simulink model "One_Sensor_Simulation"  (R2021a)
settings: Solver=FixedStepAuto  StartTime=0.0  StopTime=200  FixedStep=Ts  RelTol=1e-5
values from neighbouring files (symbols this model uses):
  accel_filter_coef = [    0.0264    0.1405    0.3331    0.3331    0.1405    0.0264]    [quad_params_ekf.m]
  g = ref_acc(3)    [ekf_measurement_jacobian.m]    (also in quad_params_ekf.m = 9.81)
  gyro_filter_den = [ 1.0000    2.2287    2.5245    1.5773    0.5410    0.0796]    [quad_params_ekf.m]
  gyro_filter_num = [ 0.2821    1.2725    2.4208    2.4208    1.2725    0.2821]    [quad_params_ekf.m]
  I = [     0.005831943165131                   0                   0 ... (first row only)    [quad_params_ekf.m]
  Kd_rates = [0.05,0.05,0.1]'    [quad_params_ekf.m]
  Kd_vel = [0.8,0.8,0.3]'    [quad_params_ekf.m]
  Ki_vel = [0.1,0.1,0.1]'    [quad_params_ekf.m]
  km = 1.2e-7    (= 1.2e-07)    [quad_params_ekf.m]
  Kp_att = [6,6,6]'    [quad_params_ekf.m]
  Kp_pos = [7,7,3]'    [quad_params_ekf.m]
  Kp_rates = [10,10,10]'    [quad_params_ekf.m]
  Kp_vel = [3,3,5]'    [quad_params_ekf.m]
  kt = 0.9e-5    (= 9e-06)    [quad_params_ekf.m]
  L = 0.2    [quad_params_ekf.m]
  m = 0.9272    [quad_params_ekf.m]
  q_init = [1;0;0;0]    [quad_params_ekf.m]
  rate_p_max = 3.5    [quad_params_ekf.m]
  thrust_max = thrust_max_per_motor*4    (= 32)    [quad_params_ekf.m]
  thrust_max_per_motor = 8    [quad_params_ekf.m]
  tilt_max = pi/6    (= 0.523598775598)    [quad_params_ekf.m]
  TQ_max_per_motor = km*(w_max.^2)    [quad_params_ekf.m]
  Ts = 0.001    [ekf_process_jacobian.m]    (also in ekf_process_model.m; quad_params_ekf.m)
  Ts_IMU = 0.001    [quad_params_ekf.m]
  Vb_init = [0;0;0]    [quad_params_ekf.m]
  vel_xy_max = 15    [quad_params_ekf.m]
  vel_z_max = 10    [quad_params_ekf.m]
  wb_init = [0;0;0]    [quad_params_ekf.m]
  Xe_init = [0;0;0]    [quad_params_ekf.m]
undefined symbols (not defined in the file or in its folder): IMU, pm_0, sigbuilder_block, Vm_0, xme_0
libraries: simulink_extras x7, aerolibutil x6, sharedutil x5, simulink x4, sharedtransform x4, pid_lib x3, aerolibcommonsys x3, aerolibnavsys x2, mspsensorlib x1, aerolibnav x1, aerolibanim x1
(part 1 of 3)
settings Model: Creator=Petronas-Tareq  LastModifiedBy=Petronas-Tareq
settings SolverCC: AutoInsertRateTranBlk=on  InsertRTBMode=Always

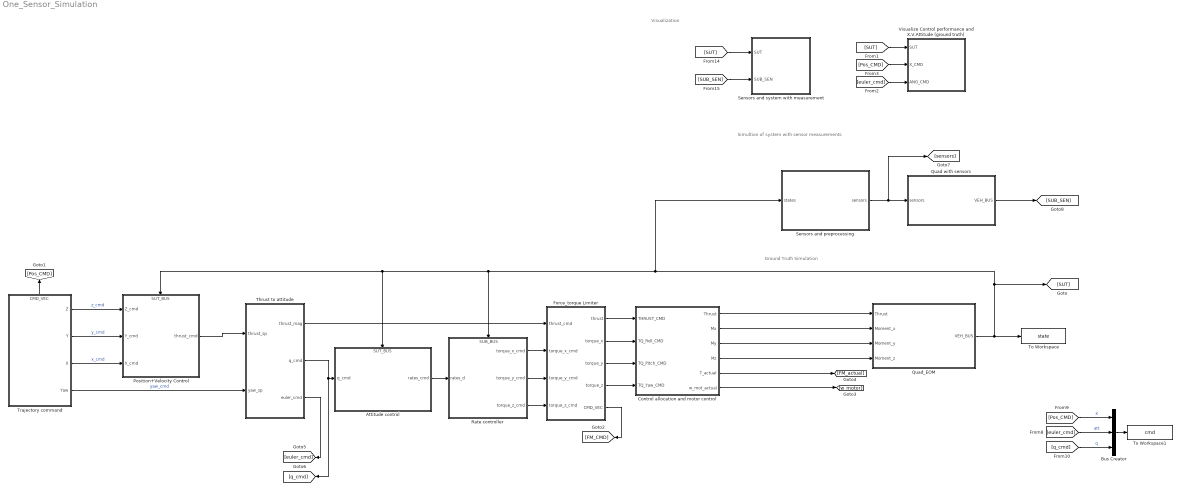
== system One_Sensor_Simulation ==
  note: Ground Truth Simulation
  note: Simultion of system with sensor measurements
  note: Visualization
  Attitude control : Subsystem
      settings: PortSchema="{\"entries\":[{\"content\":{\"sides\":[{\"content\":{\"connectorIds\":[\"In1\"]},\"type\":\"ConnectorPlacement.EquallySpacedRectSide\",\"uuid\":\"19a574f6-5314-4727-8968-5b1c9712010e\"},{\"content\":{\"connectorIds\":[\"Out1\"],\"side\":\"RIGHT\"},\"type\":\"ConnectorPlacement.EquallySpacedRectSide\",\"uuid\":\"5cd6813f-6e17-48c1-918b-7c366c6d9cfa\"},{\"content\":{\"connectorIds\":[\"In2\"],\"side\":\"TOP\"},\"type\":\"ConnectorPlacement.EquallySpacedRectSide\",\"uuid\":\"b2bca67c-c4f4-4722-89a0-a16251073bfd\"}]},\"type\":\"ConnectorPlacement.EquallySpacedConnector\",\"uuid\":\"dcbf54f5-c136-40d5-a3db-9d2776e5196c\"}],\"packageUris\":[\"http://schema.mathworks.com/mf0/Connector/R2020b\"],\"version\":\"1.0\"}"
      mask Display: image('$imagefile'); % Use "Edit Image" on toolstrip to change.
  Bus Creator : BusCreator  Inputs=3
  Control allocation and motor control : Subsystem  Variant=on  VariantControlMode=label  LabelModeActiveChoice=Choice1
      mask Display: image('$imagefile'); % Use "Edit Image" on toolstrip to change.
  Force_torque Limiter : Subsystem
  Position+Velocity Control : Subsystem
      settings: PortSchema="{\"entries\":[{\"content\":{\"sides\":[{\"content\":{\"connectorIds\":[\"In1\",\"In2\",\"In3\"]},\"type\":\"ConnectorPlacement.EquallySpacedRectSide\",\"uuid\":\"cfe37ea9-b8e2-443a-9d65-596f0fda79c9\"},{\"content\":{\"connectorIds\":[\"Out1\"],\"side\":\"RIGHT\"},\"type\":\"ConnectorPlacement.EquallySpacedRectSide\",\"uuid\":\"f39f64e1-4b16-444a-b7d2-95ecb1b2a6fa\"},{\"content\":{\"connectorIds\":[\"In4\"],\"side\":\"TOP\"},\"type\":\"ConnectorPlacement.EquallySpacedRectSide\",\"uuid\":\"52402c3a-f2ac-44cf-8c94-dbfc3f851d2b\"}]},\"type\":\"ConnectorPlacement.EquallySpacedConnector\",\"uuid\":\"0122f56a-2702-493b-af7d-a25e6b9e04ed\"}],\"packageUris\":[\"http://schema.mathworks.com/mf0/Connector/R2020b\"],\"version\":\"1.0\"}"
  Quad with sensors : Subsystem
      mask Display: image('$imagefile'); % Use "Edit Image" on toolstrip to change.
  Quad_EOM : Subsystem
      mask Display: image('$imagefile'); % Use "Edit Image" on toolstrip to change.
  Rate controller : Subsystem
      settings: PortSchema="{\"entries\":[{\"content\":{\"sides\":[{\"content\":{\"connectorIds\":[\"In1\"]},\"type\":\"ConnectorPlacement.EquallySpacedRectSide\",\"uuid\":\"0af60e35-7b10-4750-a6af-1a3d920b4771\"},{\"content\":{\"connectorIds\":[\"Out1\",\"Out2\",\"Out3\"],\"side\":\"RIGHT\"},\"type\":\"ConnectorPlacement.EquallySpacedRectSide\",\"uuid\":\"931b0f34-b3f1-4a41-949f-3d763eca3151\"},{\"content\":{\"connectorIds\":[\"In2\"],\"side\":\"TOP\"},\"type\":\"ConnectorPlacement.EquallySpacedRectSide\",\"uuid\":\"84fe42fa-07d1-4fd9-ad2f-8c6651eaa98c\"}]},\"type\":\"ConnectorPlacement.EquallySpacedConnector\",\"uuid\":\"f603d2ac-5c20-4a82-ba8b-1c7971d6778a\"}],\"packageUris\":[\"http://schema.mathworks.com/mf0/Connector/R2020b\"],\"version\":\"1.0\"}"
  Sensors and preprocessing : Subsystem
  Sensors and system with measurement : Subsystem
  Thrust to attitude : Subsystem
  To Workspace : ToWorkspace  VariableName=state  SaveFormat=Timeseries  SampleTime=-1
  To Workspace1 : ToWorkspace  VariableName=cmd  SaveFormat=Timeseries  SampleTime=-1
  Trajectory command : Subsystem  Variant=on  VariantControlMode=label  LabelModeActiveChoice=5
      settings: PortSchema="{\"entries\":[{\"content\":{\"sides\":[{\"content\":{\"connectorIds\":[]},\"type\":\"ConnectorPlacement.EquallySpacedRectSide\",\"uuid\":\"8b658e99-682c-4d99-9859-63a6cdcf875c\"},{\"content\":{\"connectorIds\":[\"Out1\",\"Out2\",\"Out3\",\"Out4\"],\"side\":\"RIGHT\"},\"type\":\"ConnectorPlacement.EquallySpacedRectSide\",\"uuid\":\"566e7e32-52b1-45cc-9bb3-5343461c1cc0\"},{\"content\":{\"connectorIds\":[\"Out5\"],\"side\":\"TOP\"},\"type\":\"ConnectorPlacement.EquallySpacedRectSide\",\"uuid\":\"4cb1ab19-6483-4408-b5f4-106b35038f17\"}]},\"type\":\"ConnectorPlacement.EquallySpacedConnector\",\"uuid\":\"dc7c82fc-432d-4c18-9829-e6c2b483f5a7\"}],\"packageUris\":[\"http://schema.mathworks.com/mf0/Connector/R2020b\"],\"version\":\"1.0\"}"
  Visualize Control performance and X,V,Attitude (ground truth) : Subsystem
  wires:
  Force_torque Limiter/5(CMD_VEC) -> [FM_CMD]
  Trajectory command/2(Y) -> Position+Velocity Control/2(Y_cmd)  "y_cmd"
  [SUT] -> Visualize Control performance and X,V,Attitude (ground truth)/1(SUT)
  [Pos_CMD] -> Visualize Control performance and X,V,Attitude (ground truth)/2(X_CMD)
  Trajectory command/3(X) -> Position+Velocity Control/3(X_cmd)  "x_cmd"
  Control allocation and motor control/1(Thrust) -> Quad_EOM/1(Thrust)
  Control allocation and motor control/2(Mx) -> Quad_EOM/2(Moment_x)
  Control allocation and motor control/3(My) -> Quad_EOM/3(Moment_y)
  Control allocation and motor control/4(Mz) -> Quad_EOM/4(Moment_z)
  Control allocation and motor control/5(T_actual) -> [FM_actual]
  Control allocation and motor control/6(w_mot_actual) -> [w_motor]
  Trajectory command/1(Z) -> Position+Velocity Control/1(Z_cmd)  "z_cmd"
  [euler_cmd] -> Visualize Control performance and X,V,Attitude (ground truth)/3(ANG_CMD)
  Force_torque Limiter/4(torque_z) -> Control allocation and motor control/4(TQ_Yaw_CMD)
  Force_torque Limiter/3(torque_y) -> Control allocation and motor control/3(TQ_Pitch_CMD)
  Force_torque Limiter/2(torque_x) -> Control allocation and motor control/2(TQ_Roll_CMD)
  Force_torque Limiter/1(thrust) -> Control allocation and motor control/1(THRUST_CMD)
  Thrust to attitude/1(thrust_mag) -> Force_torque Limiter/1(thrust_cmd)
  Rate controller/2(torque_y_cmd) -> Force_torque Limiter/3(torque_y_cmd)
  Rate controller/3(torque_z_cmd) -> Force_torque Limiter/4(torque_z_cmd)
  Rate controller/1(torque_x_cmd) -> Force_torque Limiter/2(torque_x_cmd)
  Attitude control/1(rates_cmd) -> Rate controller/1(rates_d)
  Trajectory command/5(CMD_VEC) -> [Pos_CMD]
  Bus Creator/1 -> To Workspace1/1
  [Pos_CMD] -> Bus Creator/1  "X"
  [euler_cmd] -> Bus Creator/2  "att"
  [q_cmd] -> Bus Creator/3  "q"
  Thrust to attitude/2(q_cmd) -> Attitude control/1(q_cmd), [q_cmd]
  Thrust to attitude/3(euler_cmd) -> [euler_cmd]
  Trajectory command/4(Yaw) -> Thrust to attitude/2(yaw_sp)  "yaw_cmd"
  Position+Velocity Control/1(thrust_cmd) -> Thrust to attitude/1(thrust_sp)
  Quad_EOM/1(VEH_BUS) -> Position+Velocity Control/4(SUT_BUS), Attitude control/2(SUT_BUS), Rate controller/2(SUB_BUS), Sensors and preprocessing/1(states), [SUT], To Workspace/1
  Sensors and preprocessing/1(sensors) -> [sensors], Quad with sensors/1(sensors)
  Quad with sensors/1(VEH_BUS) -> [SUB_SEN]
  [SUT] -> Sensors and system with measurement/1(SUT)
  [SUB_SEN] -> Sensors and system with measurement/2(SUB_SEN)

== system One_Sensor_Simulation/Attitude control ==
  note: Attitude control (full attitude control, i.e. yaw+thrust)
  note: Attitude Error Calculation
  q_cmd : Inport
  SUT_BUS : Inport  Port=2
  Bus Selector3 : BusSelector  OutputSignals=q
  K_attitude : Gain  Gain=Kp_att
  MATLAB Function1 : MATLAB Function  TreatAsAtomicUnit=on
  Product : Product
  Quaternion Inverse : aerolibutil/Quaternion Inverse
  Quaternion multiply : aerolibutil/Quaternion Multiplication
  Selector1 : Selector  InputPortWidth=4  IndexOptions=Index vector (dialog)  Indices=1  OutputSizes=1
  Selector2 : Selector  InputPortWidth=4  IndexOptions=Index vector (dialog)  Indices=2:4  OutputSizes=1
  k : Gain  Gain=2
  rates_cmd : Outport  VectorParamsAs1DForOutWhenUnconnected=off
  wires:
  SUT_BUS/1 -> [SUT]
  q_cmd/1 -> Quaternion multiply/2  "q_d"
  [SUT] -> Bus Selector3/1
  Bus Selector3/1 -> Quaternion Inverse/1  "<q>"
  Product/1 -> k/1  "error"
  Selector1/1 -> MATLAB Function1/1(q0)  "q0"
  MATLAB Function1/1(y) -> Product/1
  Selector2/1 -> Product/2  "q_vec"
  Quaternion multiply/1 -> Selector2/1, Selector1/1  "qe"
  k/1 -> K_attitude/1
  Quaternion Inverse/1 -> Quaternion multiply/1
  K_attitude/1 -> rates_cmd/1  "rates_cmd"

== system One_Sensor_Simulation/Control allocation and motor control ==
  note: 1) Add Subsystem or Model blocks as valid variant choices.
      | 2) You cannot connect blocks at this level. At simulation, connectivity is automatically
      | determined, based on the active variant and port name matching.
  THRUST_CMD : Inport
  TQ_Roll_CMD : Inport  Port=2
  TQ_Pitch_CMD : Inport  Port=3
  TQ_Yaw_CMD : Inport  Port=4
  Ideal Actuators with allocation : Subsystem  VariantControl=Choice2
  Ideal Actuattion (direct transfer) : Subsystem  VariantControl=Choice1
  Thrust : Outport
  Mx : Outport  Port=2
  My : Outport  Port=3
  Mz : Outport  Port=4
  T_actual : Outport  Port=5
  w_mot_actual : Outport  Port=6

== system One_Sensor_Simulation/Force_torque Limiter ==
  thrust_cmd : Inport
  torque_x_cmd : Inport  Port=2
  torque_y_cmd : Inport  Port=3
  torque_z_cmd : Inport  Port=4
  Mux : Mux
  Saturation : Saturate  UpperLimit=thrust_max  LowerLimit=-thrust_max
      settings: AttributesFormatString=|
      | MAX =    %<UpperLimit>
      | MIN = %<LowerLimit>
  Saturation1 : Saturate  UpperLimit=2*TQ_max_per_motor  LowerLimit=-2*TQ_max_per_motor
      settings: AttributesFormatString=|
      | MAX =    %<UpperLimit>
      | MIN = %<LowerLimit>
  Saturation2 : Saturate  UpperLimit=thrust_max_per_motor*L  LowerLimit=-thrust_max_per_motor *L
      settings: AttributesFormatString=|
      | MAX =    %<UpperLimit>
      | MIN = %<LowerLimit>
  Saturation3 : Saturate  UpperLimit=thrust_max_per_motor*L  LowerLimit=-thrust_max_per_motor *L
      settings: AttributesFormatString=|
      | MAX =    %<UpperLimit>
      | MIN = %<LowerLimit>
  Scope : Scope
  thrust : Outport  VectorParamsAs1DForOutWhenUnconnected=off
  torque_x : Outport  Port=2  VectorParamsAs1DForOutWhenUnconnected=off
  torque_y : Outport  Port=3  VectorParamsAs1DForOutWhenUnconnected=off
  torque_z : Outport  Port=4  VectorParamsAs1DForOutWhenUnconnected=off
  CMD_VEC : Outport  Port=5  VectorParamsAs1DForOutWhenUnconnected=off
  wires:
  torque_z_cmd/1 -> Saturation1/1
  thrust_cmd/1 -> Saturation/1
  torque_y_cmd/1 -> Saturation2/1
  torque_x_cmd/1 -> Saturation3/1
  Saturation/1 -> [THRUST], thrust/1
  Saturation3/1 -> [TQ_Roll_X], torque_x/1
  Saturation2/1 -> [TQ_Pitch_Y], torque_y/1
  Saturation1/1 -> [TQ_Yaw_Z], torque_z/1
  Mux/1 -> Scope/1, CMD_VEC/1
  [THRUST] -> Mux/1
  [TQ_Roll_X] -> Mux/2
  [TQ_Pitch_Y] -> Mux/3
  [TQ_Yaw_Z] -> Mux/4

== system One_Sensor_Simulation/Position+Velocity Control ==
  note: Velocity PID controller
  note: Position P controller
  Z_cmd : Inport
  Y_cmd : Inport  Port=2
  X_cmd : Inport  Port=3
  SUT_BUS : Inport  Port=4
  Bus Selector3 : BusSelector  OutputSignals=Xe,Ve
  Mux : Mux  Inputs=3
  Position P Controller : Subsystem
  To Workspace2 : ToWorkspace  VariableName=thrust_sp  SaveFormat=Timeseries  SampleTime=-1
  Velocity PID Controller : Subsystem
  acc setpoint : Constant  Value=[0;0;0]
  thrust_cmd : Outport
  wires:
  SUT_BUS/1 -> [SUT]
  [SUT] -> Bus Selector3/1
  Bus Selector3/1 -> [P]  "<Xe>"
  Mux/1 -> [P_sp]
  acc setpoint/1 -> [acc_sp]
  [acc_sp] -> Velocity PID Controller/3(acc_ff)  "acc_feedforwad"
  Position P Controller/1(V_sp) -> Velocity PID Controller/1(vel_cmd)  "vel_cmd"
  [P_sp] -> Position P Controller/1(pos_cmd)
  [P] -> Position P Controller/2(pos_cur)
  [V] -> Velocity PID Controller/2(vel_cur)
  Velocity PID Controller/1(thrust_sp) -> To Workspace2/1, thrust_cmd/1  "thrust_cmd"
  Bus Selector3/2 -> [V]  "<Ve>"
  Z_cmd/1 -> Mux/3
  X_cmd/1 -> Mux/1
  Y_cmd/1 -> Mux/2

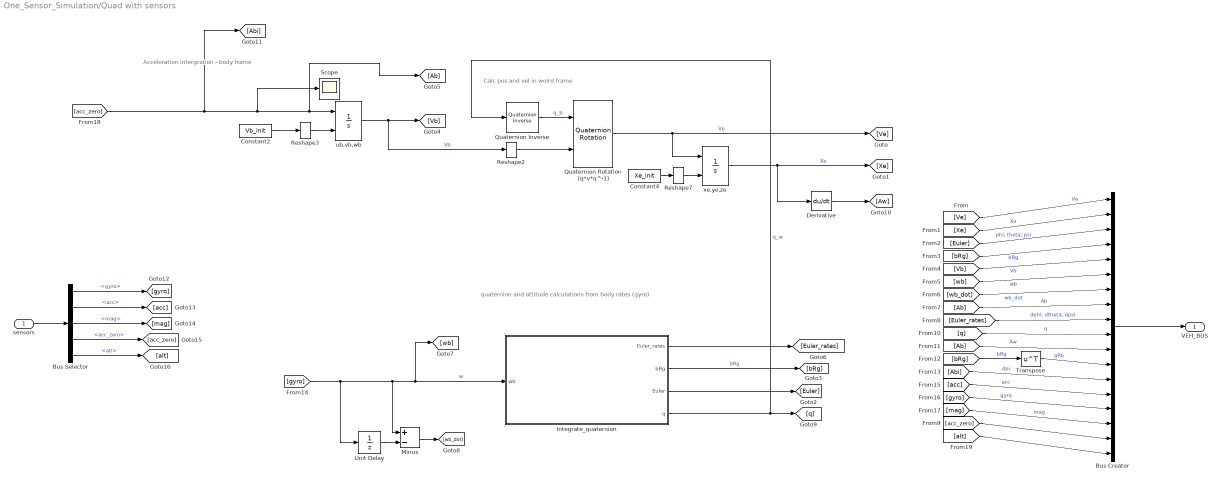
== system One_Sensor_Simulation/Quad with sensors ==
  note: Acceleration intergration - body frame
  note: Calc pos and vel in wolrd frame
  note: quaternion and attitude calculations from body rates (gyro)
  sensors : Inport
  Bus Creator : BusCreator  Inputs=18
  Bus Selector : BusSelector  OutputSignals=gyro,acc,mag,acc_zero,alt
  Constant2 : Constant  Value=Vb_init  OutDataTypeStr=Inherit: Inherit via back propagation
  Constant4 : Constant  Value=Xe_init  OutDataTypeStr=Inherit: Inherit via back propagation
  Derivative : Derivative
  Integrate_quaternion : Subsystem
  Minus : Sum  Inputs=+-
  Quaternion Inverse : aerolibutil/Quaternion Inverse
  Quaternion Rotation (q*v*q^-1) : aerolibutil/Quaternion Rotation
  Reshape2 : Reshape  OutputDimensionality=Column vector (2-D)
  Reshape3 : Reshape  OutputDimensionality=Column vector (2-D)
  Reshape7 : Reshape  OutputDimensionality=Column vector (2-D)
  Scope : Scope
  Transpose : Math  Operator=transpose  SaturateOnIntegerOverflow=on
  Unit Delay : UnitDelay  SampleTime=-1  HasFrameUpgradeWarning=on
  ub,vb,wb : Integrator  InitialConditionSource=external  InitialCondition=Vm_0
  xe,ye,ze : Integrator  InitialConditionSource=external  InitialCondition=xme_0
  VEH_BUS : Outport  VectorParamsAs1DForOutWhenUnconnected=off
  wires:
  [Euler] -> Bus Creator/3  "phi; theta; psi"
  [Xe] -> Bus Creator/2  "Xe"
  [Ve] -> Bus Creator/1  "Ve"
  [bRg] -> Bus Creator/4  "bRg"
  [Ab] -> Bus Creator/8  "Ab"
  [wb_dot] -> Bus Creator/7  "wb_dot"
  Bus Creator/1 -> VEH_BUS/1
  [Vb] -> Bus Creator/5  "Vb"
  [wb] -> Bus Creator/6  "wb"
  [Euler_rates] -> Bus Creator/9  "dphi; dtheta; dpsi"
  Constant2/1 -> Reshape3/1
  Integrate_quaternion/2(bRg) -> [bRg]  "bRg"
  Constant4/1 -> Reshape7/1
  Reshape3/1 -> ub,vb,wb/2
  Reshape7/1 -> xe,ye,ze/2
  Quaternion Rotation (q*v*q^-1)/1 -> xe,ye,ze/1, [Ve]  "Ve"
  xe,ye,ze/1 -> Derivative/1, [Xe]  "Xe"
  [gyro] -> Unit Delay/1, Minus/1, Integrate_quaternion/1(wb), [wb]  "w"
  ub,vb,wb/1 -> [Vb], Reshape2/1  "Vb"
  Integrate_quaternion/1(Euler_rates) -> [Euler_rates]
  Integrate_quaternion/3(Euler) -> [Euler]
  [q] -> Bus Creator/10  "q"
  Integrate_quaternion/4(q) -> Quaternion Inverse/1, [q]  "q_w"
  Reshape2/1 -> Quaternion Rotation (q*v*q^-1)/2
  Quaternion Inverse/1 -> Quaternion Rotation (q*v*q^-1)/1  "q_b"
  Derivative/1 -> [Aw]
  [Ab] -> Bus Creator/11  "Aw"
  [bRg] -> Transpose/1  "bRg"
  Transpose/1 -> Bus Creator/12  "gRb"
  [Abi] -> Bus Creator/13  "Abi"
  Unit Delay/1 -> Minus/2
  Minus/1 -> [wb_dot]
  Bus Selector/1 -> [gyro]  "<gyro>"
  Bus Selector/2 -> [acc]  "<acc>"
  sensors/1 -> Bus Selector/1
  [acc_zero] -> [Abi], Scope/1, [Ab], ub,vb,wb/1
  [acc] -> Bus Creator/14  "acc"
  [gyro] -> Bus Creator/15  "gyro"
  Bus Selector/3 -> [mag]  "<mag>"
  [mag] -> Bus Creator/16  "mag"
  Bus Selector/4 -> [acc_zero]  "<acc_zero>"
  [acc_zero] -> Bus Creator/17
  Bus Selector/5 -> [alt]  "<alt>"
  [alt] -> Bus Creator/18

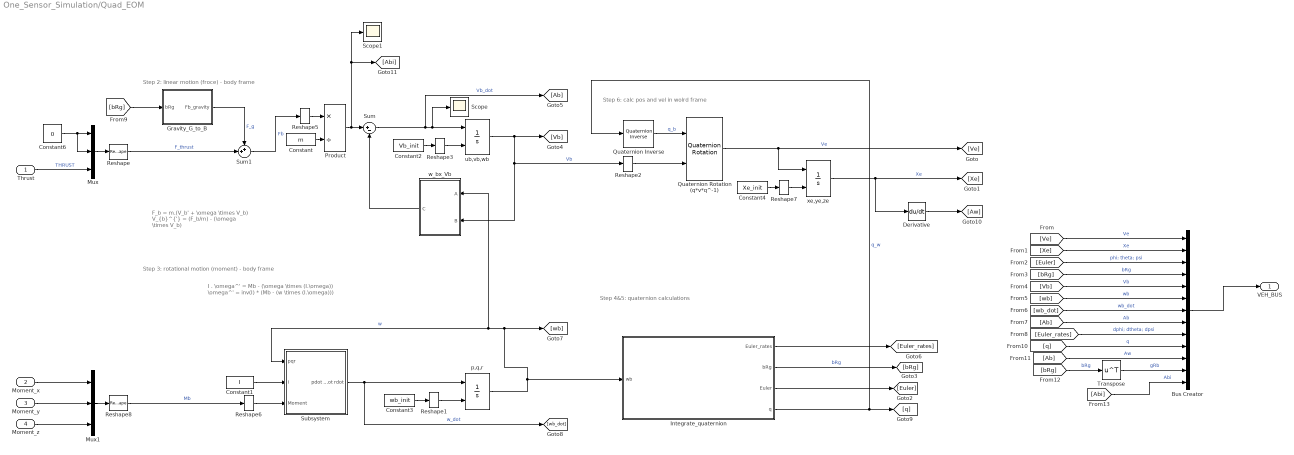
== system One_Sensor_Simulation/Quad_EOM ==
  note: Step 3: rotational motion (moment) - body frame
  note: F_b = m.(V_b' + \omega \times V_b)
      |
      | V_{b}^{'} = (F_b/m) - (\omega \times V_b)
  note: Step 2: linear motion (froce) - body frame
  note: Step 6: calc pos and vel in wolrd frame
  note: I . \omega^' = Mb - (\omega \times (I.\omega))
      |
      | \omega^' = inv(I) * (Mb - (w \times (I.\omega)))
  note: Step 4&5: quaternion calculations
  Thrust : Inport
  Moment_x : Inport  Port=2
  Moment_y : Inport  Port=3
  Moment_z : Inport  Port=4
  Bus Creator : BusCreator  Inputs=13
  Constant : Constant  Value=m  OutDataTypeStr=Inherit: Inherit via back propagation
  Constant1 : Constant  Value=I  OutDataTypeStr=Inherit: Inherit via back propagation
  Constant2 : Constant  Value=Vb_init  OutDataTypeStr=Inherit: Inherit via back propagation
  Constant3 : Constant  Value=wb_init  OutDataTypeStr=Inherit: Inherit via back propagation
  Constant4 : Constant  Value=Xe_init  OutDataTypeStr=Inherit: Inherit via back propagation
  Constant6 : Constant  Value=0
  Derivative : Derivative
  Gravity_G_to_B : Subsystem
  Integrate_quaternion : Subsystem
  Mux : Mux  Inputs=3
  Mux1 : Mux  Inputs=3
  Product : Product  Inputs=*/  SaturateOnIntegerOverflow=on  OutDataTypeStr=Inherit: Same as first input
  Quaternion Inverse : aerolibutil/Quaternion Inverse
  Quaternion Rotation (q*v*q^-1) : aerolibutil/Quaternion Rotation
  Reshape{,1..3,5..8} (8 alike) : Reshape  OutputDimensionality=Column vector (2-D)
  Scope : Scope
  Scope1 : Scope
  Subsystem : Subsystem
  Sum : Sum  Inputs=|+-  SaturateOnIntegerOverflow=on
  Sum1 : Sum  Inputs=++|
  Transpose : Math  Operator=transpose  SaturateOnIntegerOverflow=on
  "p,q,r " : Integrator  InitialConditionSource=external  InitialCondition=pm_0
  ub,vb,wb : Integrator  InitialConditionSource=external  InitialCondition=Vm_0
  w_bx_Vb : Subsystem
      mask Display:
      | text(.5,.5,'Cross\nProduct\n\nC = AxB', ...
      | 	'HorizontalAlignment','Center',...
      | 	'VerticalAlignment','middle')
  xe,ye,ze : Integrator  InitialConditionSource=external  InitialCondition=xme_0
  VEH_BUS : Outport  VectorParamsAs1DForOutWhenUnconnected=off
  wires:
  [Euler] -> Bus Creator/3  "phi; theta; psi"
  [Xe] -> Bus Creator/2  "Xe"
  [Ve] -> Bus Creator/1  "Ve"
  [bRg] -> Bus Creator/4  "bRg"
  [Ab] -> Bus Creator/8  "Ab"
  [wb_dot] -> Bus Creator/7  "wb_dot"
  Bus Creator/1 -> VEH_BUS/1
  [Vb] -> Bus Creator/5  "Vb"
  [wb] -> Bus Creator/6  "wb"
  [Euler_rates] -> Bus Creator/9  "dphi; dtheta; dpsi"
  Reshape8/1 -> Reshape6/1  "Mb"
  Reshape6/1 -> Subsystem/3(Moment)
  Reshape1/1 -> "p,q,r "/2
  Constant2/1 -> Reshape3/1
  Subsystem/1(pdot qdot rdot) -> [wb_dot], "p,q,r "/1  "w_dot"
  Constant/1 -> Product/2
  Constant1/1 -> Subsystem/2(I)
  w_bx_Vb/1(C) -> Sum/2
  Integrate_quaternion/2(bRg) -> [bRg]  "bRg"
  Sum/1 -> [Ab], Scope/1, ub,vb,wb/1  "Vb_dot"
  Constant4/1 -> Reshape7/1
  Reshape3/1 -> ub,vb,wb/2
  Reshape7/1 -> xe,ye,ze/2
  Quaternion Rotation (q*v*q^-1)/1 -> xe,ye,ze/1, [Ve]  "Ve"
  Reshape5/1 -> Product/1
  xe,ye,ze/1 -> Derivative/1, [Xe]  "Xe"
  Sum1/1 -> Reshape5/1  "Fb"
  Constant3/1 -> Reshape1/1
  Product/1 -> Scope1/1, [Abi], Sum/1
  Constant6/1 -> Mux/2, Mux/1
  Gravity_G_to_B/1(Fb_gravity) -> Sum1/1  "F_g"
  Mux/1 -> Reshape/1
  Reshape/1 -> Sum1/2  "F_thrust"
  Thrust/1 -> Mux/3  "THRUST"
  [bRg] -> Gravity_G_to_B/1(bRg)
  Moment_y/1 -> Mux1/2
  Moment_z/1 -> Mux1/3
  Mux1/1 -> Reshape8/1
  Moment_x/1 -> Mux1/1
  "p,q,r "/1 -> [wb], Subsystem/1(pqr), w_bx_Vb/1(A), Integrate_quaternion/1(wb)  "w"
  ub,vb,wb/1 -> [Vb], Reshape2/1, w_bx_Vb/2(B)  "Vb"
  Integrate_quaternion/1(Euler_rates) -> [Euler_rates]
  Integrate_quaternion/3(Euler) -> [Euler]
  [q] -> Bus Creator/10  "q"
  Integrate_quaternion/4(q) -> Quaternion Inverse/1, [q]  "q_w"
  Reshape2/1 -> Quaternion Rotation (q*v*q^-1)/2
  Quaternion Inverse/1 -> Quaternion Rotation (q*v*q^-1)/1  "q_b"
  Derivative/1 -> [Aw]
  [Ab] -> Bus Creator/11  "Aw"
  [bRg] -> Transpose/1  "bRg"
  Transpose/1 -> Bus Creator/12  "gRb"
  [Abi] -> Bus Creator/13  "Abi"

== system One_Sensor_Simulation/Rate controller ==
  note: Rate controller
  rates_d : Inport
  SUB_BUS : Inport  Port=2
  Bus Selector1 : BusSelector  OutputSignals=wb,wb_dot
  Demux : Demux  Outputs=3
  Kd_rates : Gain  Gain=Kd_rates
  Kp_rates : Gain  Gain=Kp_rates
  Scope : Scope  NumInputPorts=2
  Sum : Sum  Inputs=|+-
  Sum1 : Sum  Inputs=|+-
  limit rate p : Saturate  UpperLimit=rate_p_max  LowerLimit=-rate_p_max
  limit rate q : Saturate  UpperLimit=rate_p_max  LowerLimit=-rate_p_max
  limit rate r : Saturate  UpperLimit=rate_p_max  LowerLimit=-rate_p_max
  torque_x_cmd : Outport
  torque_y_cmd : Outport  Port=2
  torque_z_cmd : Outport  Port=3
  wires:
  Bus Selector1/2 -> Kd_rates/1  "<wb_dot>"
  Bus Selector1/1 -> Sum1/2, Scope/2  "<wb>"
  Demux/1 -> limit rate p/1
  Demux/2 -> limit rate q/1
  Demux/3 -> limit rate r/1
  SUB_BUS/1 -> Bus Selector1/1  "measurements"
  rates_d/1 -> Sum1/1, Scope/1
  Kd_rates/1 -> Sum/2  "w_d"
  Kp_rates/1 -> Sum/1
  Sum/1 -> Demux/1  "torques"
  Sum1/1 -> Kp_rates/1
  limit rate p/1 -> torque_x_cmd/1
  limit rate q/1 -> torque_y_cmd/1
  limit rate r/1 -> torque_z_cmd/1

== system One_Sensor_Simulation/Sensors and preprocessing ==
  states : Inport
  Bus Creator4 : BusCreator  Inputs=5
  IMU+altitude : Subsystem
  Memory1 : Memory  InheritSampleTime=on
  Preprocessing and Filtering : Subsystem
  Scope : Scope
  Scope1 : Scope
  sensors : Outport
  wires:
  states/1 -> Memory1/1
  Bus Creator4/1 -> sensors/1
  IMU+altitude/1(acc) -> Scope/1, Preprocessing and Filtering/1(acc_raw)  "acc_raw"
  IMU+altitude/2(gyro) -> Scope1/1, Preprocessing and Filtering/2(gyro_raw)  "gyro_raw"
  Memory1/1 -> IMU+altitude/1(States)
  IMU+altitude/3(alt) -> Preprocessing and Filtering/3(alt_raw)  "alt_raw"
  IMU+altitude/4(mag) -> Preprocessing and Filtering/4(mag_raw)  "mag_raw"
  Preprocessing and Filtering/1(acc_zero) -> Bus Creator4/1  "acc_zero"
  Preprocessing and Filtering/2(acc) -> Bus Creator4/2  "acc"
  Preprocessing and Filtering/3(gyro) -> Bus Creator4/3  "gyro"
  Preprocessing and Filtering/4(alt) -> Bus Creator4/4  "alt"
  Preprocessing and Filtering/5(mag) -> Bus Creator4/5  "mag"

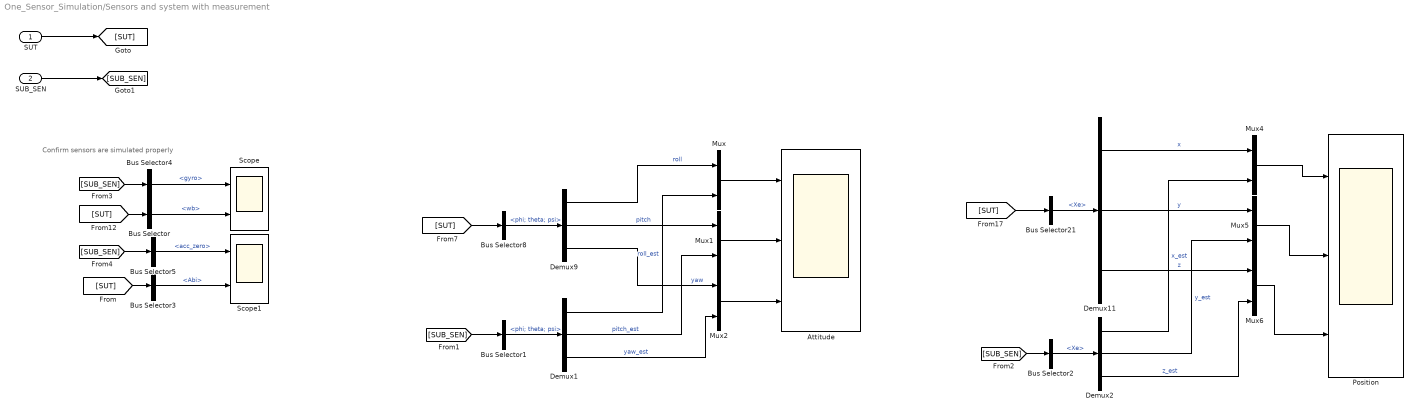
== system One_Sensor_Simulation/Sensors and system with measurement ==
  note: Confirm sensors are simulated properly
  SUT : Inport
  SUB_SEN : Inport  Port=2
  "Attitude " : Scope  NumInputPorts=3
  Bus Selector : BusSelector  OutputSignals=wb
  Bus Selector1 : BusSelector  OutputSignals=phi; theta; psi
  Bus Selector2 : BusSelector  OutputSignals=Xe
  Bus Selector21 : BusSelector  OutputSignals=Xe
  Bus Selector3 : BusSelector  OutputSignals=Abi
  Bus Selector4 : BusSelector  OutputSignals=gyro
  Bus Selector5 : BusSelector  OutputSignals=acc_zero
  Bus Selector8 : BusSelector  OutputSignals=phi; theta; psi
  Demux{1..2,9,11} (4 alike) : Demux  Outputs=3
  Mux{,1..2,4..6} (6 alike) : Mux  Inputs=2
  Position : Scope  NumInputPorts=3
  Scope : Scope  NumInputPorts=2
  Scope1 : Scope  NumInputPorts=2
  wires:
  Mux4/1 -> Position/1
  Demux11/2 -> Mux5/1  "y"
  [SUT] -> Bus Selector21/1
  Demux11/1 -> Mux4/1  "x"
  Mux5/1 -> Position/2
  Demux11/3 -> Mux6/1  "z"
  Bus Selector21/1 -> Demux11/1  "<Xe>"
  [SUT] -> Bus Selector8/1
  Mux6/1 -> Position/3
  Bus Selector8/1 -> Demux9/1  "<phi; theta; psi>"
  Mux2/1 -> "Attitude "/3
  Demux9/2 -> Mux1/1  "pitch"
  Demux9/3 -> Mux2/1  "yaw"
  Mux1/1 -> "Attitude "/2
  Mux/1 -> "Attitude "/1
  Demux9/1 -> Mux/1  "roll"
  SUT/1 -> [SUT]
  SUB_SEN/1 -> [SUB_SEN]
  [SUB_SEN] -> Bus Selector1/1
  Bus Selector1/1 -> Demux1/1  "<phi; theta; psi>"
  Demux1/1 -> Mux/2  "roll_est"
  Demux1/2 -> Mux1/2  "pitch_est"
  Demux1/3 -> Mux2/2  "yaw_est"
  [SUB_SEN] -> Bus Selector2/1
  Bus Selector2/1 -> Demux2/1  "<Xe>"
  Demux2/1 -> Mux4/2  "x_est"
  Demux2/2 -> Mux5/2  "y_est"
  Demux2/3 -> Mux6/2  "z_est"
  Bus Selector/1 -> Scope/2  "<wb>"
  Bus Selector4/1 -> Scope/1  "<gyro>"
  Bus Selector5/1 -> Scope1/1  "<acc_zero>"
  [SUT] -> Bus Selector3/1
  [SUB_SEN] -> Bus Selector4/1
  [SUB_SEN] -> Bus Selector5/1
  [SUT] -> Bus Selector/1
  Bus Selector3/1 -> Scope1/2  "<Abi>"

== system One_Sensor_Simulation/Thrust to attitude ==
  note: Thrust vector and Yaw to Attitude and total Thrust
  thrust_sp : Inport
  yaw_sp : Inport  Port=2
  Bus Creator : BusCreator  Inputs=3
  Demux4 : Demux  Outputs=3
  Direction Cosine Matrix to Quaternions : sharedtransform/Direction Cosine Matrix  to Quaternions  aMode=0  action=None  tolerance=eps(2)
      settings: SourceProductBaseCode=AE,PW,DR,MT,UV,VE
  MATLAB Function4 : MATLAB Function  TreatAsAtomicUnit=on
  Quaternions to Rotation Angles : sharedtransform/Quaternions to Rotation Angles  rotationOrder=ZYX  aMode=aMode
      settings: SourceProductBaseCode=AE,PW,DR,MT,UV,VE
  Scope1 : Scope
  Scope2 : Scope
  To Workspace : ToWorkspace  VariableName=thrust_unit_dir  SaveFormat=Timeseries  SampleTime=-1
  To Workspace1 : ToWorkspace  VariableName=thrust_mag  SaveFormat=Timeseries  SampleTime=-1
  thrust_mag : Outport
  q_cmd : Outport  Port=2
  euler_cmd : Outport  Port=3
  wires:
  thrust_sp/1 -> Scope1/1, MATLAB Function4/1(thrust_sp)  "thrust_cmd"
  MATLAB Function4/1(R_sp) -> To Workspace/1, Direction Cosine Matrix to Quaternions/1
  MATLAB Function4/2(thrust_mag) -> thrust_mag/1, To Workspace1/1
  Direction Cosine Matrix to Quaternions/1 -> q_cmd/1, Quaternions to Rotation Angles/1
  yaw_sp/1 -> MATLAB Function4/2(yaw_sp)  "yaw_cmd"
  Demux4/1 -> Bus Creator/1  "yaw"
  Demux4/3 -> Bus Creator/3  "roll"
  Bus Creator/1 -> Scope2/1, euler_cmd/1
  Demux4/2 -> Bus Creator/2  "pitch"
  Quaternions to Rotation Angles/1 -> Demux4/1

== system One_Sensor_Simulation/Trajectory command ==
  Altitude : Subsystem  VariantControl=1
  Ground : Subsystem  VariantControl=0
  Position Trajectory : Subsystem  VariantControl=5
  Test to visualize thrust dir : Subsystem  VariantControl=6
  X Sine : Subsystem  VariantControl=4
  X ramp : Subsystem  VariantControl=9
  X square : Subsystem  VariantControl=7
  Y Sine : Subsystem  VariantControl=3
  Y ramp : Subsystem  VariantControl=8
  Yaw Sine : Subsystem  VariantControl=2
  Yaw steps : Subsystem  VariantControl=10
  Z : Outport
  Y : Outport  Port=2
  X : Outport  Port=3
  Yaw : Outport  Port=4
  CMD_VEC : Outport  Port=5

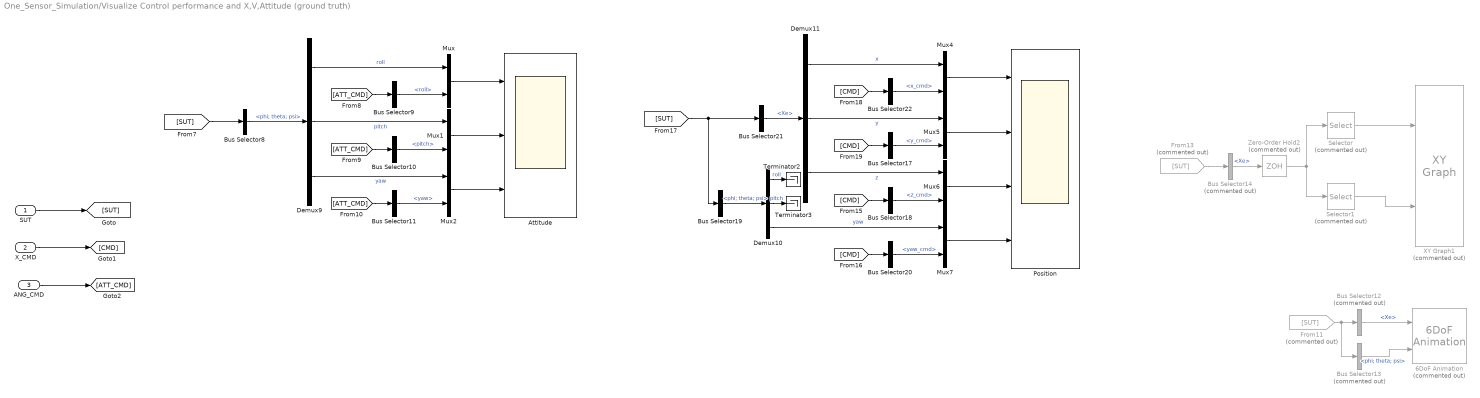
== system One_Sensor_Simulation/Visualize Control performance and X,V,Attitude (ground truth) ==
  SUT : Inport
  X_CMD : Inport  Port=2
  ANG_CMD : Inport  Port=3
  6DoF Animation : aerolibanim/6DoF Animation  Commented=on  u1=[-20 20 -20 20 -20 20]  u2=0.05  u3=0.5  u4=[-5 -5 0 5]  u5=Fly alongside  u6=[0 0 0]  u7=10  u8=on
  "Attitude " : Scope  NumInputPorts=3
  Bus Selector10 : BusSelector  OutputSignals=pitch
  Bus Selector11 : BusSelector  OutputSignals=yaw
  Bus Selector12 : BusSelector  Commented=on  OutputSignals=Xe
  Bus Selector13 : BusSelector  Commented=on  OutputSignals=phi; theta; psi
  Bus Selector14 : BusSelector  Commented=on  OutputSignals=Xe
  Bus Selector17 : BusSelector  OutputSignals=y_cmd
  Bus Selector18 : BusSelector  OutputSignals=z_cmd
  Bus Selector19 : BusSelector  OutputSignals=phi; theta; psi
  Bus Selector20 : BusSelector  OutputSignals=yaw_cmd
  Bus Selector21 : BusSelector  OutputSignals=Xe
  Bus Selector22 : BusSelector  OutputSignals=x_cmd
  Bus Selector8 : BusSelector  OutputSignals=phi; theta; psi
  Bus Selector9 : BusSelector  OutputSignals=roll
  Demux10 : Demux  Outputs=3
  Demux11 : Demux  Outputs=3
  Demux9 : Demux  Outputs=3
  From11 : From  Commented=on  GotoTag=SUT
  From13 : From  Commented=on  GotoTag=SUT
  Mux{,1..2,4..7} (7 alike) : Mux  Inputs=2
  Position : Scope  NumInputPorts=4
  Selector : Selector  Commented=on  InputPortWidth=3  IndexOptions=Index vector (dialog)  Indices=1  OutputSizes=1
  Selector1 : Selector  Commented=on  InputPortWidth=3  IndexOptions=Index vector (dialog)  Indices=2  OutputSizes=1
  Terminator2 : Terminator
  Terminator3 : Terminator
  XY Graph1 : simulink/Sinks/XY Graph  Commented=on  xmin=-1  xmax=30  ymin=-1  ymax=35  st=-1
  Zero-Order Hold2 : ZeroOrderHold  Commented=on  SampleTime=0.1
  wires:
  SUT/1 -> [SUT]
  X_CMD/1 -> [CMD]
  [SUT] -> Bus Selector8/1
  Demux9/2 -> Mux1/1  "pitch"
  Demux9/1 -> Mux/1  "roll"
  Bus Selector8/1 -> Demux9/1  "<phi; theta; psi>"
  Mux/1 -> "Attitude "/1
  Mux1/1 -> "Attitude "/2
  Mux2/1 -> "Attitude "/3
  Demux9/3 -> Mux2/1  "yaw"
  [ATT_CMD] -> Bus Selector9/1
  Bus Selector9/1 -> Mux/2  "<roll>"
  [ATT_CMD] -> Bus Selector10/1
  Bus Selector10/1 -> Mux1/2  "<pitch>"
  [ATT_CMD] -> Bus Selector11/1
  Bus Selector11/1 -> Mux2/2  "<yaw>"
  From13/1 -> Bus Selector14/1
  Bus Selector14/1 -> Zero-Order Hold2/1  "<Xe>"
  Zero-Order Hold2/1 -> Selector1/1, Selector/1
  Demux10/3 -> Mux7/1  "yaw"
  Mux7/1 -> Position/4
  Demux11/1 -> Mux4/1  "x"
  [CMD] -> Bus Selector20/1
  Bus Selector20/1 -> Mux7/2  "<yaw_cmd>"
  [CMD] -> Bus Selector17/1
  [SUT] -> Bus Selector21/1, Bus Selector19/1
  Demux10/2 -> Terminator3/1  "pitch"
  Mux6/1 -> Position/3
  Bus Selector19/1 -> Demux10/1  "<phi; theta; psi>"
  Demux10/1 -> Terminator2/1  "roll"
  Demux11/2 -> Mux5/1  "y"
  Bus Selector17/1 -> Mux5/2  "<y_cmd>"
  Mux4/1 -> Position/1
  Demux11/3 -> Mux6/1  "z"
  [CMD] -> Bus Selector22/1
  Mux5/1 -> Position/2
  Bus Selector22/1 -> Mux4/2  "<x_cmd>"
  Bus Selector18/1 -> Mux6/2  "<z_cmd>"
  [CMD] -> Bus Selector18/1
  Bus Selector21/1 -> Demux11/1  "<Xe>"
  ANG_CMD/1 -> [ATT_CMD]
  Selector/1 -> XY Graph1/1
  Selector1/1 -> XY Graph1/2
  From11/1 -> Bus Selector13/1, Bus Selector12/1
  Bus Selector12/1 -> 6DoF Animation/1  "<Xe>"
  Bus Selector13/1 -> 6DoF Animation/2  "<phi; theta; psi>"

== system One_Sensor_Simulation/Control allocation and motor control/Ideal Actuators with allocation ==
  THRUST_CMD : Inport
  TQ_Roll_CMD : Inport  Port=2
  TQ_Pitch_CMD : Inport  Port=3
  TQ_Yaw_CMD : Inport  Port=4
  Control allocation : Subsystem
  Perfect actuators : Subsystem  VariantControl=Choice2
  Thrust : Outport
  Mx : Outport  Port=2
  My : Outport  Port=3
  Mz : Outport  Port=4
  T_actual : Outport  Port=5
  w_mot_actual : Outport  Port=6
  wires:
  Control allocation/1(w_command) -> Perfect actuators/1(w_cmd)
  THRUST_CMD/1 -> Control allocation/1(THRUST_CMD)
  TQ_Pitch_CMD/1 -> Control allocation/3(TQ_Pitch_CMD)
  TQ_Roll_CMD/1 -> Control allocation/2(TQ_Roll_CMD)
  TQ_Yaw_CMD/1 -> Control allocation/4(TQ_Yaw_CMD)
  Perfect actuators/5(T_actual) -> T_actual/1
  Perfect actuators/6(w_mot_actual) -> w_mot_actual/1
  Perfect actuators/3(My) -> My/1
  Perfect actuators/2(Mx) -> Mx/1
  Perfect actuators/4(Mz) -> Mz/1
  Perfect actuators/1(Thrust) -> Thrust/1

== system One_Sensor_Simulation/Control allocation and motor control/Ideal Actuattion (direct transfer) ==
  THRUST_CMD : Inport
  TQ_Roll_CMD : Inport  Port=2
  TQ_Pitch_CMD : Inport  Port=3
  TQ_Yaw_CMD : Inport  Port=4
  Mux : Mux
  Zero : Constant  Value=[0;0;0;0]  OutDataTypeStr=Inherit: Inherit via back propagation
  Thrust : Outport
  Mx : Outport  Port=2
  My : Outport  Port=3
  Mz : Outport  Port=4
  T_actual : Outport  Port=5
  w_mot_actual : Outport  Port=6
  wires:
  Zero/1 -> w_mot_actual/1
  TQ_Pitch_CMD/1 -> Mux/3, My/1
  TQ_Roll_CMD/1 -> Mux/2, Mx/1
  TQ_Yaw_CMD/1 -> Mux/4, Mz/1
  THRUST_CMD/1 -> Mux/1, Thrust/1
  Mux/1 -> T_actual/1

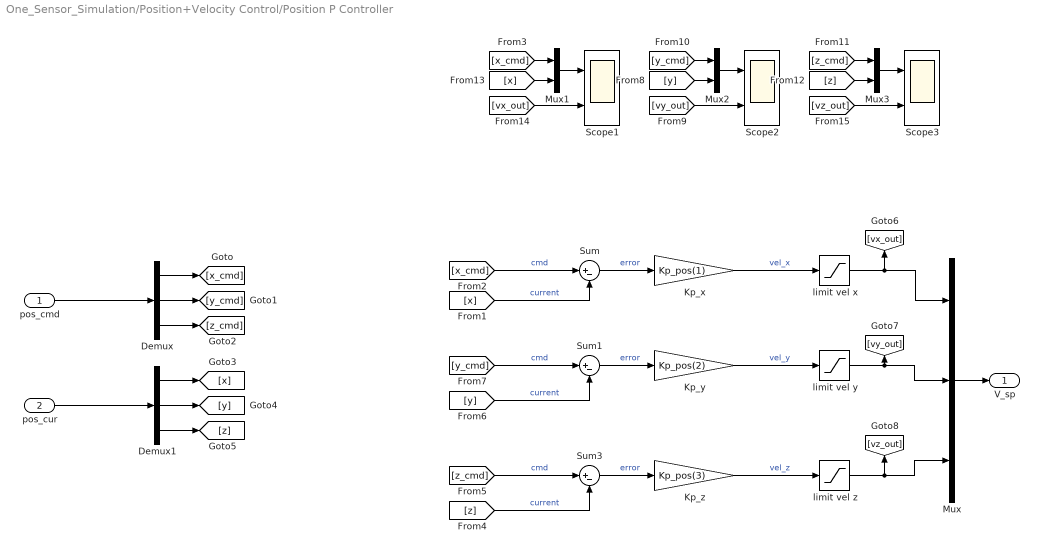
== system One_Sensor_Simulation/Position+Velocity Control/Position P Controller ==
  pos_cmd : Inport
  pos_cur : Inport  Port=2
  Demux : Demux  Outputs=3
  Demux1 : Demux  Outputs=3
  Kp_x : Gain  Gain=Kp_pos(1)
  Kp_y : Gain  Gain=Kp_pos(2)
  Kp_z : Gain  Gain=Kp_pos(3)
  Mux : Mux  Inputs=3
  Mux1 : Mux  Inputs=2
  Mux2 : Mux  Inputs=2
  Mux3 : Mux  Inputs=2
  Scope1 : Scope  NumInputPorts=2
  Scope2 : Scope  NumInputPorts=2
  Scope3 : Scope  NumInputPorts=2
  Sum : Sum  Inputs=|+-
  Sum1 : Sum  Inputs=|+-
  Sum3 : Sum  Inputs=|+-
  limit vel x : Saturate  UpperLimit=vel_xy_max  LowerLimit=-vel_xy_max
  limit vel y : Saturate  UpperLimit=vel_xy_max  LowerLimit=-vel_xy_max
  limit vel z : Saturate  UpperLimit=vel_z_max  LowerLimit=-vel_z_max
  V_sp : Outport
  wires:
  pos_cmd/1 -> Demux/1
  pos_cur/1 -> Demux1/1
  Demux/1 -> [x_cmd]
  Demux/2 -> [y_cmd]
  Demux/3 -> [z_cmd]
  Demux1/1 -> [x]
  Demux1/3 -> [z]
  Demux1/2 -> [y]
  [x_cmd] -> Sum/1  "cmd"
  Sum/1 -> Kp_x/1  "error"
  Mux/1 -> V_sp/1
  Kp_x/1 -> limit vel x/1  "vel_x"
  [x] -> Sum/2  "current"
  [z_cmd] -> Sum3/1  "cmd"
  [z] -> Sum3/2  "current"
  Sum3/1 -> Kp_z/1  "error"
  [y_cmd] -> Sum1/1  "cmd"
  [y] -> Sum1/2  "current"
  Sum1/1 -> Kp_y/1  "error"
  Kp_z/1 -> limit vel z/1  "vel_z"
  limit vel x/1 -> [vx_out], Mux/1
  Kp_y/1 -> limit vel y/1  "vel_y"
  limit vel y/1 -> [vy_out], Mux/2
  limit vel z/1 -> [vz_out], Mux/3
  [x_cmd] -> Mux1/1
  Mux1/1 -> Scope1/1
  [vx_out] -> Scope1/2
  [x] -> Mux1/2
  [y_cmd] -> Mux2/1
  Mux2/1 -> Scope2/1
  [vy_out] -> Scope2/2
  [y] -> Mux2/2
  [z_cmd] -> Mux3/1
  Mux3/1 -> Scope3/1
  [vz_out] -> Scope3/2
  [z] -> Mux3/2

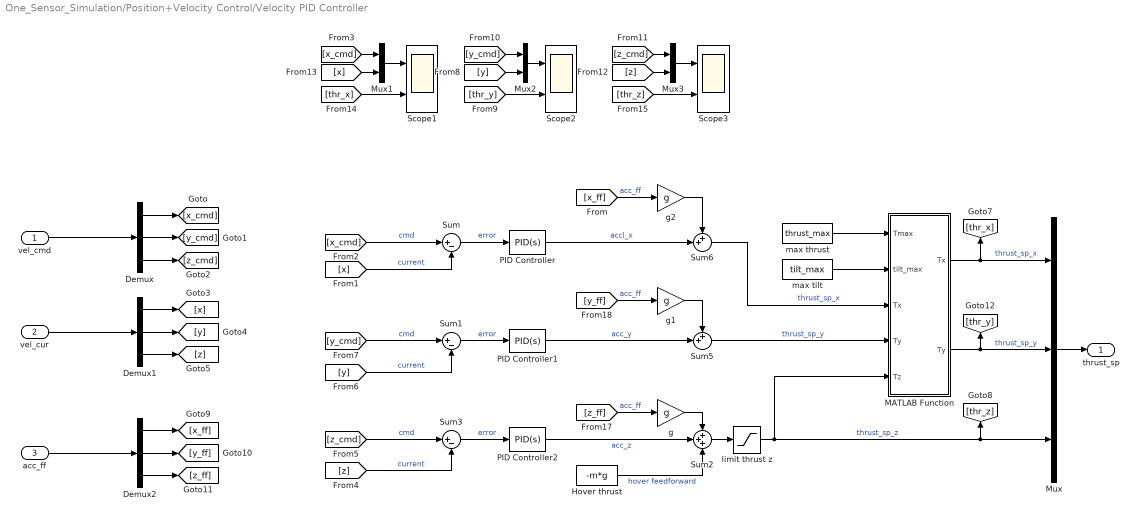
== system One_Sensor_Simulation/Position+Velocity Control/Velocity PID Controller ==
  vel_cmd : Inport
  vel_cur : Inport  Port=2
  acc_ff : Inport  Port=3
  Demux : Demux  Outputs=3
  Demux1 : Demux  Outputs=3
  Demux2 : Demux  Outputs=3
  Hover thrust : Constant  Value=-m*g
  MATLAB Function : MATLAB Function  TreatAsAtomicUnit=on
  Mux : Mux  Inputs=3
  Mux1 : Mux  Inputs=2
  Mux2 : Mux  Inputs=2
  Mux3 : Mux  Inputs=2
  PID Controller : pid_lib/PID Controller  Controller=PID  Form=Parallel  TimeDomain=Continuous-time  UseExternalTs=off  SampleTime=-1  IntegratorMethod=Forward Euler  FilterMethod=Forward Euler  ControllerParametersSource=internal  P=Kp_vel(1)  I=Ki_vel(1)  D=Kd_vel(1)  UseFilter=on  N=100  TunerSelectOption=Transfer Function Based (PID Tuner App)  InitialConditionSource=internal  InitialConditionForIntegrator=0  InitialConditionForFilter=0  DifferentiatorICPrevScaledInput=0  ExternalReset=none  TrackingMode=off  Kt=1  LimitOutput=off  SatLimitsSource=internal  UpperSaturationLimit=inf  LowerSaturationLimit=-inf  LinearizeAsGain=on  AntiWindupMode=none  Kb=1  POutMin=[]  POutMax=[]  IOutMin=[]  IOutMax=[]  DOutMin=[]  DOutMax=[]  NOutMin=[]  NOutMax=[]  SumOutMin=[]  SumOutMax=[]  SaturationOutMin=[]  SaturationOutMax=[]  PParamMin=[]  PParamMax=[]  IParamMin=[]  IParamMax=[]  DParamMin=[]  DParamMax=[]  NParamMin=[]  NParamMax=[]  KbParamMin=[]  KbParamMax=[]  KtParamMin=[]  KtParamMax=[]  KbOutMin=[]  KbOutMax=[]  KtOutMin=[]  KtOutMax=[]  IntegratorOutMin=[]  IntegratorOutMax=[]  FilterOutMin=[]  FilterOutMax=[]  SumI1OutMin=[]  SumI1OutMax=[]  SumI2OutMin=[]  SumI2OutMax=[]  SumI3OutMin=[]  SumI3OutMax=[]  SumI4OutMin=[]  SumI4OutMax=[]  SumDOutMin=[]  SumDOutMax=[]  DifferentiatorOutMin=[]  DifferentiatorOutMax=[]  FilterDiffOutCoefMin=[]  FilterDiffOutCoefMax=[]  ReciprocalOutMin=[]  ReciprocalOutMax=[]  SumDenOutMin=[]  SumDenOutMax=[]  SumNumOutMin=[]  SumNumOutMax=[]  DivideOutMin=[]  DivideOutMax=[]  UdiffTsProdOutMin=[]  UdiffTsProdOutMax=[]  NTsProdOutMin=[]  NTsProdOutMax=[]  UintegralTsProdOutMin=[]  UintegralTsProdOutMax=[]  UngainTsProdOutMin=[]  UngainTsProdOutMax=[]  IntegratorContinuousStateAttributes=''  IntegratorStateMustResolveToSignalObject=off  IntegratorRTWStateStorageClass=Auto  FilterContinuousStateAttributes=''  FilterStateMustResolveToSignalObject=off  FilterRTWStateStorageClass=Auto  ParallelPVariant=InternalParameters  IdealPVariant=Disabled  IVariant=InternalParameters  DVariant=InternalParameters  IntegratorVariant=Continuous  SatVariant=Disabled  AWVariant=Passthrough  PCopyVariant=Disabled  TRVariant=Disabled  FdbkBlocksVariant=Forward  IdealPFdbkVariant=Disabled  SatFdbkVariant=Disabled  DerivativeFilterVariant=ContFilter  NVariant=InternalParameters  NCopyVariant=Disabled  FilterICVariant=InternalICsFilter  IntegratorICVariant=InternalICs  ExternalResetVariant=Disabled  TRSumVariant=Passthrough  SumFdbkVariant=Disabled  SumVariant=Sum_PID  TsampFilterVariant=InternalTs  TsampNgainVariant=Passthrough  TsampIntegralVariant=Passthrough  ExternalSaturationOutDataTypeStr=Inherit: Same as second input
  PID Controller1 : pid_lib/PID Controller  Controller=PID  Form=Parallel  TimeDomain=Continuous-time  UseExternalTs=off  SampleTime=-1  IntegratorMethod=Forward Euler  FilterMethod=Forward Euler  ControllerParametersSource=internal  P=Kp_vel(2)  I=Ki_vel(2)  D=Kd_vel(2)  UseFilter=on  N=100  TunerSelectOption=Transfer Function Based (PID Tuner App)  InitialConditionSource=internal  InitialConditionForIntegrator=0  InitialConditionForFilter=0  DifferentiatorICPrevScaledInput=0  ExternalReset=none  TrackingMode=off  Kt=1  LimitOutput=off  SatLimitsSource=internal  UpperSaturationLimit=inf  LowerSaturationLimit=-inf  LinearizeAsGain=on  AntiWindupMode=none  Kb=1  POutMin=[]  POutMax=[]  IOutMin=[]  IOutMax=[]  DOutMin=[]  DOutMax=[]  NOutMin=[]  NOutMax=[]  SumOutMin=[]  SumOutMax=[]  SaturationOutMin=[]  SaturationOutMax=[]  PParamMin=[]  PParamMax=[]  IParamMin=[]  IParamMax=[]  DParamMin=[]  DParamMax=[]  NParamMin=[]  NParamMax=[]  KbParamMin=[]  KbParamMax=[]  KtParamMin=[]  KtParamMax=[]  KbOutMin=[]  KbOutMax=[]  KtOutMin=[]  KtOutMax=[]  IntegratorOutMin=[]  IntegratorOutMax=[]  FilterOutMin=[]  FilterOutMax=[]  SumI1OutMin=[]  SumI1OutMax=[]  SumI2OutMin=[]  SumI2OutMax=[]  SumI3OutMin=[]  SumI3OutMax=[]  SumI4OutMin=[]  SumI4OutMax=[]  SumDOutMin=[]  SumDOutMax=[]  DifferentiatorOutMin=[]  DifferentiatorOutMax=[]  FilterDiffOutCoefMin=[]  FilterDiffOutCoefMax=[]  ReciprocalOutMin=[]  ReciprocalOutMax=[]  SumDenOutMin=[]  SumDenOutMax=[]  SumNumOutMin=[]  SumNumOutMax=[]  DivideOutMin=[]  DivideOutMax=[]  UdiffTsProdOutMin=[]  UdiffTsProdOutMax=[]  NTsProdOutMin=[]  NTsProdOutMax=[]  UintegralTsProdOutMin=[]  UintegralTsProdOutMax=[]  UngainTsProdOutMin=[]  UngainTsProdOutMax=[]  IntegratorContinuousStateAttributes=''  IntegratorStateMustResolveToSignalObject=off  IntegratorRTWStateStorageClass=Auto  FilterContinuousStateAttributes=''  FilterStateMustResolveToSignalObject=off  FilterRTWStateStorageClass=Auto  ParallelPVariant=InternalParameters  IdealPVariant=Disabled  IVariant=InternalParameters  DVariant=InternalParameters  IntegratorVariant=Continuous  SatVariant=Disabled  AWVariant=Passthrough  PCopyVariant=Disabled  TRVariant=Disabled  FdbkBlocksVariant=Forward  IdealPFdbkVariant=Disabled  SatFdbkVariant=Disabled  DerivativeFilterVariant=ContFilter  NVariant=InternalParameters  NCopyVariant=Disabled  FilterICVariant=InternalICsFilter  IntegratorICVariant=InternalICs  ExternalResetVariant=Disabled  TRSumVariant=Passthrough  SumFdbkVariant=Disabled  SumVariant=Sum_PID  TsampFilterVariant=InternalTs  TsampNgainVariant=Passthrough  TsampIntegralVariant=Passthrough  ExternalSaturationOutDataTypeStr=Inherit: Same as second input
  PID Controller2 : pid_lib/PID Controller  Controller=PID  Form=Parallel  TimeDomain=Continuous-time  UseExternalTs=off  SampleTime=-1  IntegratorMethod=Forward Euler  FilterMethod=Forward Euler  ControllerParametersSource=internal  P=Kp_vel(3)  I=Ki_vel(3)  D=Kd_vel(3)  UseFilter=on  N=100  TunerSelectOption=Transfer Function Based (PID Tuner App)  InitialConditionSource=internal  InitialConditionForIntegrator=0  InitialConditionForFilter=0  DifferentiatorICPrevScaledInput=0  ExternalReset=none  TrackingMode=off  Kt=1  LimitOutput=off  SatLimitsSource=internal  UpperSaturationLimit=inf  LowerSaturationLimit=-inf  LinearizeAsGain=on  AntiWindupMode=none  Kb=1  POutMin=[]  POutMax=[]  IOutMin=[]  IOutMax=[]  DOutMin=[]  DOutMax=[]  NOutMin=[]  NOutMax=[]  SumOutMin=[]  SumOutMax=[]  SaturationOutMin=[]  SaturationOutMax=[]  PParamMin=[]  PParamMax=[]  IParamMin=[]  IParamMax=[]  DParamMin=[]  DParamMax=[]  NParamMin=[]  NParamMax=[]  KbParamMin=[]  KbParamMax=[]  KtParamMin=[]  KtParamMax=[]  KbOutMin=[]  KbOutMax=[]  KtOutMin=[]  KtOutMax=[]  IntegratorOutMin=[]  IntegratorOutMax=[]  FilterOutMin=[]  FilterOutMax=[]  SumI1OutMin=[]  SumI1OutMax=[]  SumI2OutMin=[]  SumI2OutMax=[]  SumI3OutMin=[]  SumI3OutMax=[]  SumI4OutMin=[]  SumI4OutMax=[]  SumDOutMin=[]  SumDOutMax=[]  DifferentiatorOutMin=[]  DifferentiatorOutMax=[]  FilterDiffOutCoefMin=[]  FilterDiffOutCoefMax=[]  ReciprocalOutMin=[]  ReciprocalOutMax=[]  SumDenOutMin=[]  SumDenOutMax=[]  SumNumOutMin=[]  SumNumOutMax=[]  DivideOutMin=[]  DivideOutMax=[]  UdiffTsProdOutMin=[]  UdiffTsProdOutMax=[]  NTsProdOutMin=[]  NTsProdOutMax=[]  UintegralTsProdOutMin=[]  UintegralTsProdOutMax=[]  UngainTsProdOutMin=[]  UngainTsProdOutMax=[]  IntegratorContinuousStateAttributes=''  IntegratorStateMustResolveToSignalObject=off  IntegratorRTWStateStorageClass=Auto  FilterContinuousStateAttributes=''  FilterStateMustResolveToSignalObject=off  FilterRTWStateStorageClass=Auto  ParallelPVariant=InternalParameters  IdealPVariant=Disabled  IVariant=InternalParameters  DVariant=InternalParameters  IntegratorVariant=Continuous  SatVariant=Disabled  AWVariant=Passthrough  PCopyVariant=Disabled  TRVariant=Disabled  FdbkBlocksVariant=Forward  IdealPFdbkVariant=Disabled  SatFdbkVariant=Disabled  DerivativeFilterVariant=ContFilter  NVariant=InternalParameters  NCopyVariant=Disabled  FilterICVariant=InternalICsFilter  IntegratorICVariant=InternalICs  ExternalResetVariant=Disabled  TRSumVariant=Passthrough  SumFdbkVariant=Disabled  SumVariant=Sum_PID  TsampFilterVariant=InternalTs  TsampNgainVariant=Passthrough  TsampIntegralVariant=Passthrough  ExternalSaturationOutDataTypeStr=Inherit: Same as second input
  Scope1 : Scope  NumInputPorts=2
  Scope2 : Scope  NumInputPorts=2
  Scope3 : Scope  NumInputPorts=2
  Sum : Sum  Inputs=|+-
  Sum1 : Sum  Inputs=|+-
  Sum2 : Sum  Inputs=+++
  Sum3 : Sum  Inputs=|+-
  Sum5 : Sum  Inputs=++|
  Sum6 : Sum  Inputs=++|
  g : Gain  Gain=g
  g1 : Gain  Gain=g
  g2 : Gain  Gain=g
  limit thrust z : Saturate  UpperLimit=thrust_max  LowerLimit=-thrust_max
  max thrust : Constant  Value=thrust_max
  max tilt : Constant  Value=tilt_max
  thrust_sp : Outport
  wires:
  vel_cmd/1 -> Demux/1
  vel_cur/1 -> Demux1/1
  Demux/1 -> [x_cmd]
  Demux/2 -> [y_cmd]
  Demux/3 -> [z_cmd]
  Demux1/1 -> [x]
  Demux1/3 -> [z]
  Demux1/2 -> [y]
  [x_cmd] -> Sum/1  "cmd"
  [thr_x] -> Scope1/2
  Sum/1 -> PID Controller/1  "error"
  Mux/1 -> thrust_sp/1
  [x] -> Sum/2  "current"
  [z_cmd] -> Sum3/1  "cmd"
  [z] -> Sum3/2  "current"
  Sum3/1 -> PID Controller2/1  "error"
  [y_cmd] -> Sum1/1  "cmd"
  [y] -> Sum1/2  "current"
  Sum1/1 -> PID Controller1/1  "error"
  limit thrust z/1 -> [thr_z], Mux/3, MATLAB Function/5(Tz)  "thrust_sp_z"
  Demux2/3 -> [z_ff]
  acc_ff/1 -> Demux2/1
  Demux2/2 -> [y_ff]
  Demux2/1 -> [x_ff]
  Hover thrust/1 -> Sum2/3  "hover feedforward"
  PID Controller2/1 -> Sum2/2  "acc_z"
  [z_ff] -> g/1  "acc_ff"
  g/1 -> Sum2/1
  [y_ff] -> g1/1  "acc_ff"
  PID Controller1/1 -> Sum5/2  "acc_y"
  g1/1 -> Sum5/1
  g2/1 -> Sum6/1
  [x_ff] -> g2/1  "acc_ff"
  PID Controller/1 -> Sum6/2  "accl_x"
  Sum2/1 -> limit thrust z/1
  max thrust/1 -> MATLAB Function/1(Tmax)
  max tilt/1 -> MATLAB Function/2(tilt_max)
  Mux1/1 -> Scope1/1
  [x_cmd] -> Mux1/1
  [x] -> Mux1/2
  [y_cmd] -> Mux2/1
  Mux2/1 -> Scope2/1
  [thr_y] -> Scope2/2
  [y] -> Mux2/2
  [z_cmd] -> Mux3/1
  Mux3/1 -> Scope3/1
  [thr_z] -> Scope3/2
  [z] -> Mux3/2
  MATLAB Function/1(Tx) -> Mux/1, [thr_x]  "thrust_sp_x"
  Sum6/1 -> MATLAB Function/3("Tx ")  "thrust_sp_x"
  Sum5/1 -> MATLAB Function/4("Ty ")  "thrust_sp_y"
  MATLAB Function/2(Ty) -> [thr_y], Mux/2  "thrust_sp_y"

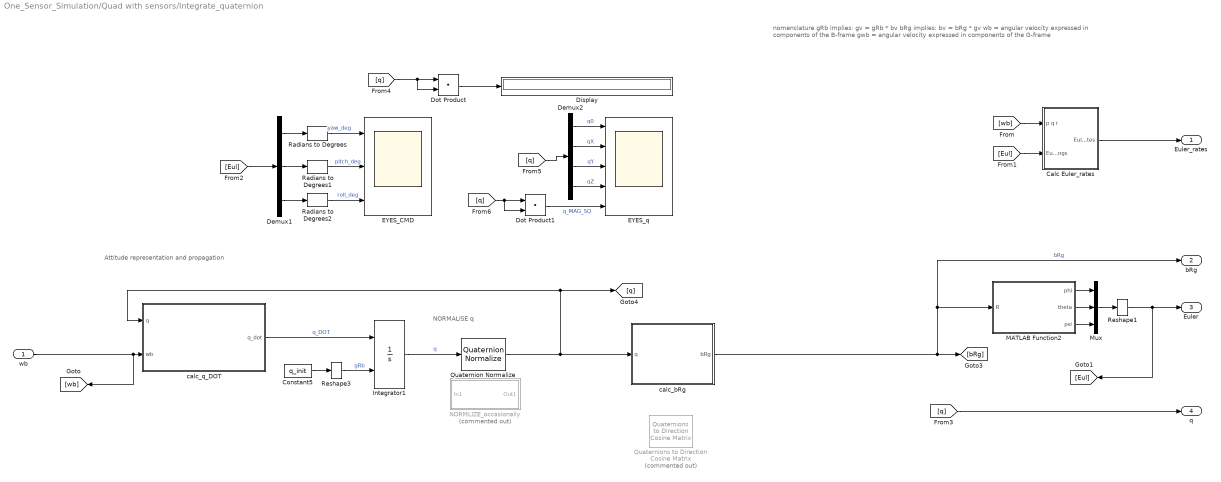
== system One_Sensor_Simulation/Quad with sensors/Integrate_quaternion ==
  note: Attitude representation and propagation
  note: nomenclature
      | gRb implies: gv = gRb * bv
      | bRg implies: bv = bRg * gv
      |
      | wb = angular velocity expressed in components of the B-frame
      | gwb = angular velocity expressed in components of the G-frame
  note: NORMALISE q
  wb : Inport
  Calc Euler_rates : Subsystem
  Constant5 : Constant  Value=q_init  OutDataTypeStr=Inherit: Inherit via back propagation
  Demux1 : Demux  Outputs=3
  Demux2 : Demux
  Display : Display
  Dot Product : DotProduct  InputSameDT=on  OutDataTypeStr=Inherit: Inherit via internal rule
  Dot Product1 : DotProduct  InputSameDT=on  OutDataTypeStr=Inherit: Inherit via internal rule
  EYES_CMD : Scope  NumInputPorts=3
  EYES_q : Scope  NumInputPorts=5
  Integrator1 : Integrator  InitialConditionSource=external
  MATLAB Function2 : MATLAB Function  TreatAsAtomicUnit=on
  Mux : Mux  Inputs=3
  NORMLIZE_occasionally : Subsystem  Commented=on
  Quaternion Normalize : sharedutil/Quaternion Normalize  aMode=aMode
      settings: SourceProductBaseCode=AE,PW,DR,MT,UV,VE
  Quaternions to Direction Cosine Matrix : sharedtransform/Quaternions to  Direction Cosine Matrix  Commented=on  aMode=aMode
      settings: SourceProductBaseCode=AE,PW,DR,MT,UV,VE
  Radians to Degrees : simulink_extras/Transformations/Radians to Degrees
  Radians to Degrees1 : simulink_extras/Transformations/Radians to Degrees
  Radians to Degrees2 : simulink_extras/Transformations/Radians to Degrees
  Reshape1 : Reshape  OutputDimensionality=Column vector (2-D)
  Reshape3 : Reshape  OutputDimensionality=Column vector (2-D)
  calc_bRg : MATLAB Function  TreatAsAtomicUnit=on
  calc_q_DOT : MATLAB Function  TreatAsAtomicUnit=on
  Euler_rates : Outport
  bRg : Outport  Port=2
  Euler : Outport  Port=3
  q : Outport  Port=4
  wires:
  Calc Euler_rates/1(Euler_rates) -> Euler_rates/1
  [Eul] -> Demux1/1
  Demux1/2 -> Radians to Degrees1/1
  Demux1/3 -> Radians to Degrees2/1
  Radians to Degrees2/1 -> EYES_CMD/3  "roll_deg"
  Radians to Degrees1/1 -> EYES_CMD/2  "pitch_deg"
  Radians to Degrees/1 -> EYES_CMD/1  "yaw_deg"
  Demux1/1 -> Radians to Degrees/1
  [Eul] -> Calc Euler_rates/2(Euler_angs)
  [wb] -> Calc Euler_rates/1("p q r ")
  Reshape1/1 -> [Eul], Euler/1
  Mux/1 -> Reshape1/1
  MATLAB Function2/3(psi) -> Mux/3
  MATLAB Function2/2(theta) -> Mux/2
  MATLAB Function2/1(phi) -> Mux/1
  Demux2/3 -> EYES_q/3  "qY"
  [q] -> Demux2/1
  Demux2/2 -> EYES_q/2  "qX"
  Demux2/1 -> EYES_q/1  "q0"
  [q] -> Dot Product1/2, Dot Product1/1
  Demux2/4 -> EYES_q/4  "qZ"
  Dot Product1/1 -> EYES_q/5  "q_MAG_SQ"
  Dot Product/1 -> Display/1
  [q] -> Dot Product/2, Dot Product/1
  Integrator1/1 -> Quaternion Normalize/1  "q"
  Quaternion Normalize/1 -> calc_bRg/1(q), [q], calc_q_DOT/1(q)
  calc_bRg/1(bRg) -> bRg/1, MATLAB Function2/1(R), [bRg]  "bRg"
  calc_q_DOT/1(q_dot) -> Integrator1/1  "q_DOT"
  Constant5/1 -> Reshape3/1
  wb/1 -> calc_q_DOT/2(wb), [wb]
  Reshape3/1 -> Integrator1/2  "gRb"
  [q] -> q/1

== system One_Sensor_Simulation/Quad_EOM/Gravity_G_to_B ==
  note: F_B = ^BR_G * F_G
  bRg : Inport
  Product : Product  Multiplication=Matrix(*)
  Product1 : Product
  gravity vector in inertial frame : Constant  Value=[0;0;g]  VectorParams1D=off
  mass : Constant  Value=m
  Fb_gravity : Outport  VectorParamsAs1DForOutWhenUnconnected=off
  wires:
  bRg/1 -> Product/1
  Product/1 -> Fb_gravity/1  "F_garvity in body frame"
  Product1/1 -> Product/2  "m*g"
  gravity vector in inertial frame/1 -> Product1/1  "Fg"
  mass/1 -> Product1/2
